simulink subsystem "Comb_Slip"  (R2021b)
settings: Solver=VariableStepAuto  StartTime=0.0  StopTime=10.0  RelTol=1e-3
undefined symbols (not defined in the file): a_f, afx_f, agx_f, agy_f, mu_tire_F
settings Model: Creator=tsuyoshi  LastModifiedBy=tsuyoshi

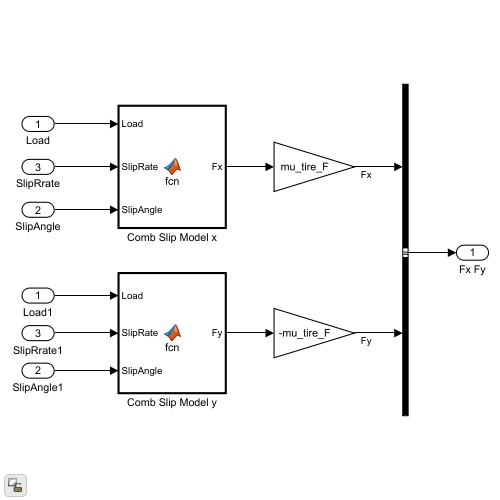
[thumbnail: Simulink's stored preview of the top-level diagram]
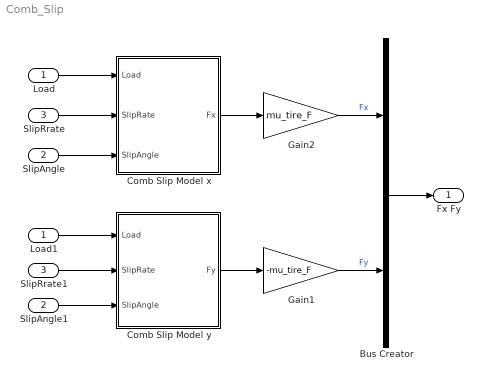
== system Comb_Slip ==
  Load : Inport
  SlipAngle : Inport  Port=2
  SlipRrate : Inport  Port=3
  Bus Creator : BusCreator  Inputs=2
  Comb Slip Model x : MATLAB Function  TreatAsAtomicUnit=on
  Comb Slip Model y : MATLAB Function  TreatAsAtomicUnit=on
  Gain1 : Gain  Gain=-mu_tire_F
  Gain2 : Gain  Gain=mu_tire_F
  Load1 : InportShadow
  SlipAngle1 : InportShadow  Port=2
  SlipRrate1 : InportShadow  Port=3
  Fx Fy : Outport
  wires:
  Load/1 -> Comb Slip Model x/1(Load)
  SlipRrate/1 -> Comb Slip Model x/2(SlipRate)
  SlipAngle/1 -> Comb Slip Model x/3(SlipAngle)
  Comb Slip Model x/1(Fx) -> Gain2/1
  Gain2/1 -> Bus Creator/1  "Fx"
  Gain1/1 -> Bus Creator/2  "Fy"
  Comb Slip Model y/1(Fy) -> Gain1/1
  SlipRrate1/1 -> Comb Slip Model y/2(SlipRate)
  Load1/1 -> Comb Slip Model y/1(Load)
  SlipAngle1/1 -> Comb Slip Model y/3(SlipAngle)
  Bus Creator/1 -> Fx Fy/1

== matlab function Comb_Slip/Comb Slip Model x ==
  data: Load input; SlipRate input; Fx output; SlipAngle input; agx_f parameter; afx_f parameter
function Fx = fcn(Load, SlipRate, SlipAngle, agx_f, afx_f)
    C = agx_f(1);
    D = fcnPureFx(Load, SlipRate, afx_f);
    if D==0
        D=eps;
    end
    E = Load*agx_f(4) + agx_f(5);
    B = agx_f(2)*sin(2*atan(Load/agx_f(3)))/(D*C);
    Fx = D*cos(C*atan(B*SlipAngle-E*(B*SlipAngle-atan(B*SlipAngle))));
end

function PureFx = fcnPureFx(Load, SlipRate, afx_f)
    C = afx_f(1);
    D = (Load*afx_f(2) + afx_f(3))*Load;
    E = Load*afx_f(6) + afx_f(7);
    B = afx_f(4)*sin(2*atan(Load/afx_f(5)))/(D*C);
    PureFx = D*sin(C*atan(B*SlipRate-E*(B*SlipRate-atan(B*SlipRate))));
end

== matlab function Comb_Slip/Comb Slip Model y ==
  data: Load input; Fy output; SlipRate input; SlipAngle input; agy_f parameter; a_f parameter
function Fy = fcn(Load, SlipRate, SlipAngle, agy_f, a_f)
    C = agy_f(1);
    D = fcnPureFy(Load, SlipAngle, a_f);
    if D==0
        D=eps;
    end
    E = Load*agy_f(4) + agy_f(5);
    B = agy_f(2)*sin(2*atan(Load/agy_f(3)))/(D*C);
    Fy = D*cos(C*atan(B*SlipRate-E*(B*SlipRate-atan(B*SlipRate))));
end

function PureFy = fcnPureFy(Load, SlipAngle, a_f)
    C = a_f(1);
    D = (Load*a_f(2) + a_f(3))*Load;
    E = Load*a_f(6) + a_f(7);
    B = a_f(4)*sin(2*atan(Load/a_f(5)))/(D*C);
    PureFy = D*sin(C*atan(B*SlipAngle-E*(B*SlipAngle-atan(B*SlipAngle))));
end
